simulink library "TOWER_MASTER"  (Simulink 8.8)
settings: Solver=ode45  StartTime=0.0  StopTime=10.0  RelTol=1e-3  EnableMultiTasking=on
undefined symbols (not defined in the file): AC, AC2THRESHOLD, BF_WD_MASTER, GAS_WD_MASTER, GASAC, SIXOSEM_F_WD_AC_MASTER
libraries: cdsEpicsOut x163, cdsFilt x111, cdsTP x68, cdsFiltCtrl x56, cdsEpicsIn x47, cdsMuxMatrix x14, cdsRms x14, TOWER_MASTER x11, STATE_BIO_MASTER x8, cdsEpicsBinIn x6, cdsFunctionCall x4, VIS_LIB x2
(part 18 of 19)

== system TOWER_MASTER/common_blocks/OKUTOMIGASMODAL/TEST ==
  Ground{1..5} (5 alike) : Ground
  M1 : cdsFilt/Subsystem  Tag=cdsFilt  Description=|
      | Purpose:                                                                                                                                                                                                                                  
      | Standard CDS IIR filter module.                                                                                                                                                                                                           
      |                                                                                                                                                                                                                                           
      | Operation:                                                                                                                                                                                                                                
      | Consists of 10 second order section IIR filters, plus a ramped gain stage. In FE code, also provides pre-defined test points and excitation channel inputs. The filter coefficients are defined in the LIGO system using the 'foton' tool.
      |                                                                                                                                                                                                                                           
      | Usage:                                                                                                                                                                                                                                    
      | Name the part with the desired filter module name.
      settings: AttributesFormatString=%<Tag>
  M2 : cdsFilt/Subsystem  Tag=cdsFilt  Description=|
      | Purpose:                                                                                                                                                                                                                                  
      | Standard CDS IIR filter module.                                                                                                                                                                                                           
      |                                                                                                                                                                                                                                           
      | Operation:                                                                                                                                                                                                                                
      | Consists of 10 second order section IIR filters, plus a ramped gain stage. In FE code, also provides pre-defined test points and excitation channel inputs. The filter coefficients are defined in the LIGO system using the 'foton' tool.
      |                                                                                                                                                                                                                                           
      | Usage:                                                                                                                                                                                                                                    
      | Name the part with the desired filter module name.
      settings: AttributesFormatString=%<Tag>
  M3 : cdsFilt/Subsystem  Tag=cdsFilt  Description=|
      | Purpose:                                                                                                                                                                                                                                  
      | Standard CDS IIR filter module.                                                                                                                                                                                                           
      |                                                                                                                                                                                                                                           
      | Operation:                                                                                                                                                                                                                                
      | Consists of 10 second order section IIR filters, plus a ramped gain stage. In FE code, also provides pre-defined test points and excitation channel inputs. The filter coefficients are defined in the LIGO system using the 'foton' tool.
      |                                                                                                                                                                                                                                           
      | Usage:                                                                                                                                                                                                                                    
      | Name the part with the desired filter module name.
      settings: AttributesFormatString=%<Tag>
  M4 : cdsFilt/Subsystem  Tag=cdsFilt  Description=|
      | Purpose:                                                                                                                                                                                                                                  
      | Standard CDS IIR filter module.                                                                                                                                                                                                           
      |                                                                                                                                                                                                                                           
      | Operation:                                                                                                                                                                                                                                
      | Consists of 10 second order section IIR filters, plus a ramped gain stage. In FE code, also provides pre-defined test points and excitation channel inputs. The filter coefficients are defined in the LIGO system using the 'foton' tool.
      |                                                                                                                                                                                                                                           
      | Usage:                                                                                                                                                                                                                                    
      | Name the part with the desired filter module name.
      settings: AttributesFormatString=%<Tag>
  M5 : cdsFilt/Subsystem  Tag=cdsFilt  Description=|
      | Purpose:                                                                                                                                                                                                                                  
      | Standard CDS IIR filter module.                                                                                                                                                                                                           
      |                                                                                                                                                                                                                                           
      | Operation:                                                                                                                                                                                                                                
      | Consists of 10 second order section IIR filters, plus a ramped gain stage. In FE code, also provides pre-defined test points and excitation channel inputs. The filter coefficients are defined in the LIGO system using the 'foton' tool.
      |                                                                                                                                                                                                                                           
      | Usage:                                                                                                                                                                                                                                    
      | Name the part with the desired filter module name.
      settings: AttributesFormatString=%<Tag>
  M1_Out : Outport
  M2_Out : Outport  Port=2
  M3_Out : Outport  Port=3
  M4_Out : Outport  Port=4
  M5_Out : Outport  Port=5
  wires:
  Ground5/1 -> M5/1
  Ground4/1 -> M4/1
  M4/1 -> M4_Out/1
  M5/1 -> M5_Out/1
  Ground3/1 -> M3/1
  Ground2/1 -> M2/1
  Ground1/1 -> M1/1
  M1/1 -> M1_Out/1
  M2/1 -> M2_Out/1
  M3/1 -> M3_Out/1

== system TOWER_MASTER/common_blocks/OKUTOMIKALMAN/ADD_OUTPUT ==
  D_In1 : Inport
  D_In2 : Inport  Port=2
  D_In3 : Inport  Port=3
  D_In4 : Inport  Port=4
  D_In5 : Inport  Port=5
  D_In6 : Inport  Port=6
  C_In1 : Inport  Port=7
  C_In2 : Inport  Port=8
  C_In3 : Inport  Port=9
  C_In4 : Inport  Port=10
  C_In5 : Inport  Port=11
  C_In6 : Inport  Port=12
  Sum{1..6} (6 alike) : Sum
  Xest_Out1 : Outport
  Xest_Out2 : Outport  Port=2
  Xest_Out3 : Outport  Port=3
  Xest_Out4 : Outport  Port=4
  Xest_Out5 : Outport  Port=5
  Xest_Out6 : Outport  Port=6
  wires:
  Sum1/1 -> Xest_Out1/1
  Sum2/1 -> Xest_Out2/1
  Sum3/1 -> Xest_Out3/1
  Sum4/1 -> Xest_Out4/1
  Sum5/1 -> Xest_Out5/1
  Sum6/1 -> Xest_Out6/1
  C_In1/1 -> Sum1/1
  C_In2/1 -> Sum2/1
  C_In3/1 -> Sum3/1
  C_In4/1 -> Sum4/1
  C_In6/1 -> Sum6/1
  C_In5/1 -> Sum5/1
  D_In1/1 -> Sum1/2
  D_In6/1 -> Sum6/2
  D_In5/1 -> Sum5/2
  D_In4/1 -> Sum4/2
  D_In3/1 -> Sum3/2
  D_In2/1 -> Sum2/2

== system TOWER_MASTER/common_blocks/OKUTOMIKALMAN/ADD_STATE ==
  B_In1 : Inport
  B_In2 : Inport  Port=2
  B_In3 : Inport  Port=3
  B_In4 : Inport  Port=4
  B_In5 : Inport  Port=5
  B_In6 : Inport  Port=6
  A_In1 : Inport  Port=7
  A_In2 : Inport  Port=8
  A_In3 : Inport  Port=9
  A_In4 : Inport  Port=10
  A_In5 : Inport  Port=11
  A_In6 : Inport  Port=12
  Sum{1..6} (6 alike) : Sum
  dX_Out1 : Outport
  dX_Out2 : Outport  Port=2
  dX_Out3 : Outport  Port=3
  dX_Out4 : Outport  Port=4
  dX_Out5 : Outport  Port=5
  dX_Out6 : Outport  Port=6
  wires:
  B_In2/1 -> Sum2/2
  B_In3/1 -> Sum3/2
  B_In4/1 -> Sum4/2
  B_In5/1 -> Sum5/2
  B_In6/1 -> Sum6/2
  B_In1/1 -> Sum1/2
  A_In5/1 -> Sum5/1
  A_In6/1 -> Sum6/1
  A_In4/1 -> Sum4/1
  A_In3/1 -> Sum3/1
  A_In2/1 -> Sum2/1
  A_In1/1 -> Sum1/1
  Sum6/1 -> dX_Out6/1
  Sum5/1 -> dX_Out5/1
  Sum4/1 -> dX_Out4/1
  Sum3/1 -> dX_Out3/1
  Sum2/1 -> dX_Out2/1
  Sum1/1 -> dX_Out1/1

== system TOWER_MASTER/common_blocks/OKUTOMIKALMAN/KEST ==
  X1_In : Inport
  X2_In : Inport  Port=2
  X3_In : Inport  Port=3
  X4_In : Inport  Port=4
  X5_In : Inport  Port=5
  X6_In : Inport  Port=6
  X1 : cdsFilt/Subsystem  Tag=cdsFilt  Description=|
      | Purpose:                                                                                                                                                                                                                                  
      | Standard CDS IIR filter module.                                                                                                                                                                                                           
      |                                                                                                                                                                                                                                           
      | Operation:                                                                                                                                                                                                                                
      | Consists of 10 second order section IIR filters, plus a ramped gain stage. In FE code, also provides pre-defined test points and excitation channel inputs. The filter coefficients are defined in the LIGO system using the 'foton' tool.
      |                                                                                                                                                                                                                                           
      | Usage:                                                                                                                                                                                                                                    
      | Name the part with the desired filter module name.
      settings: AttributesFormatString=%<Tag>
  X2 : cdsFilt/Subsystem  Tag=cdsFilt  Description=|
      | Purpose:                                                                                                                                                                                                                                  
      | Standard CDS IIR filter module.                                                                                                                                                                                                           
      |                                                                                                                                                                                                                                           
      | Operation:                                                                                                                                                                                                                                
      | Consists of 10 second order section IIR filters, plus a ramped gain stage. In FE code, also provides pre-defined test points and excitation channel inputs. The filter coefficients are defined in the LIGO system using the 'foton' tool.
      |                                                                                                                                                                                                                                           
      | Usage:                                                                                                                                                                                                                                    
      | Name the part with the desired filter module name.
      settings: AttributesFormatString=%<Tag>
  X3 : cdsFilt/Subsystem  Tag=cdsFilt  Description=|
      | Purpose:                                                                                                                                                                                                                                  
      | Standard CDS IIR filter module.                                                                                                                                                                                                           
      |                                                                                                                                                                                                                                           
      | Operation:                                                                                                                                                                                                                                
      | Consists of 10 second order section IIR filters, plus a ramped gain stage. In FE code, also provides pre-defined test points and excitation channel inputs. The filter coefficients are defined in the LIGO system using the 'foton' tool.
      |                                                                                                                                                                                                                                           
      | Usage:                                                                                                                                                                                                                                    
      | Name the part with the desired filter module name.
      settings: AttributesFormatString=%<Tag>
  X4 : cdsFilt/Subsystem  Tag=cdsFilt  Description=|
      | Purpose:                                                                                                                                                                                                                                  
      | Standard CDS IIR filter module.                                                                                                                                                                                                           
      |                                                                                                                                                                                                                                           
      | Operation:                                                                                                                                                                                                                                
      | Consists of 10 second order section IIR filters, plus a ramped gain stage. In FE code, also provides pre-defined test points and excitation channel inputs. The filter coefficients are defined in the LIGO system using the 'foton' tool.
      |                                                                                                                                                                                                                                           
      | Usage:                                                                                                                                                                                                                                    
      | Name the part with the desired filter module name.
      settings: AttributesFormatString=%<Tag>
  X5 : cdsFilt/Subsystem  Tag=cdsFilt  Description=|
      | Purpose:                                                                                                                                                                                                                                  
      | Standard CDS IIR filter module.                                                                                                                                                                                                           
      |                                                                                                                                                                                                                                           
      | Operation:                                                                                                                                                                                                                                
      | Consists of 10 second order section IIR filters, plus a ramped gain stage. In FE code, also provides pre-defined test points and excitation channel inputs. The filter coefficients are defined in the LIGO system using the 'foton' tool.
      |                                                                                                                                                                                                                                           
      | Usage:                                                                                                                                                                                                                                    
      | Name the part with the desired filter module name.
      settings: AttributesFormatString=%<Tag>
  X6 : cdsFilt/Subsystem  Tag=cdsFilt  Description=|
      | Purpose:                                                                                                                                                                                                                                  
      | Standard CDS IIR filter module.                                                                                                                                                                                                           
      |                                                                                                                                                                                                                                           
      | Operation:                                                                                                                                                                                                                                
      | Consists of 10 second order section IIR filters, plus a ramped gain stage. In FE code, also provides pre-defined test points and excitation channel inputs. The filter coefficients are defined in the LIGO system using the 'foton' tool.
      |                                                                                                                                                                                                                                           
      | Usage:                                                                                                                                                                                                                                    
      | Name the part with the desired filter module name.
      settings: AttributesFormatString=%<Tag>
  X1_Out : Outport
  X2_Out : Outport  Port=2
  X3_Out : Outport  Port=3
  X4_Out : Outport  Port=4
  X5_Out : Outport  Port=5
  X6_Out : Outport  Port=6
  wires:
  X2_In/1 -> X2/1
  X1_In/1 -> X1/1
  X6_In/1 -> X6/1
  X2/1 -> X2_Out/1
  X1/1 -> X1_Out/1
  X6/1 -> X6_Out/1
  X5_In/1 -> X5/1
  X4_In/1 -> X4/1
  X3_In/1 -> X3/1
  X5/1 -> X5_Out/1
  X4/1 -> X4_Out/1
  X3/1 -> X3_Out/1

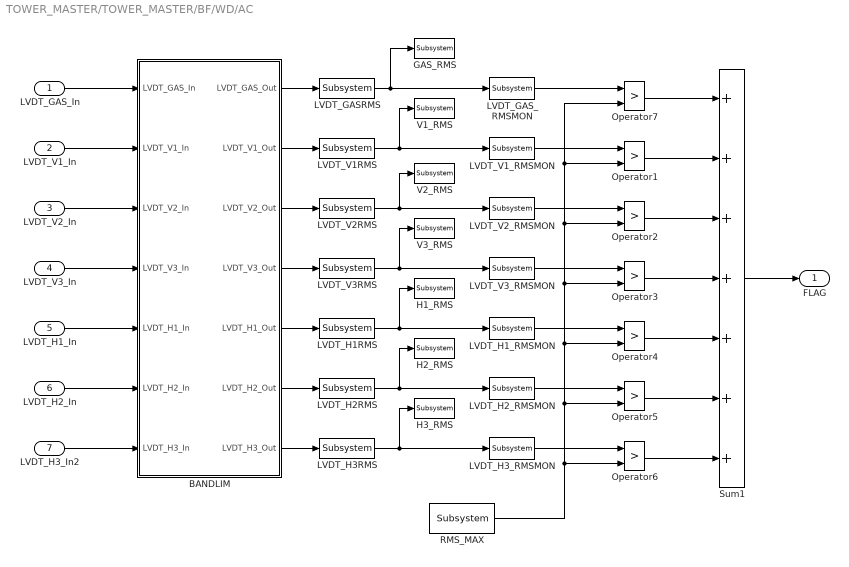
== system TOWER_MASTER/TOWER_MASTER/BF/WD/AC ==
  LVDT_GAS_In : Inport
  LVDT_V1_In : Inport  Port=2
  LVDT_V2_In : Inport  Port=3
  LVDT_V3_In : Inport  Port=4
  LVDT_H1_In : Inport  Port=5
  LVDT_H2_In : Inport  Port=6
  LVDT_H3_In2 : Inport  Port=7
  BANDLIM : Subsystem
  GAS_RMS : cdsTP/Subsystem  Tag=Test Point
      settings: AttributesFormatString=%<Tag>
  H1_RMS : cdsTP/Subsystem  Tag=Test Point
      settings: AttributesFormatString=%<Tag>
  H2_RMS : cdsTP/Subsystem  Tag=Test Point
      settings: AttributesFormatString=%<Tag>
  H3_RMS : cdsTP/Subsystem  Tag=Test Point
      settings: AttributesFormatString=%<Tag>
  LVDT_GASRMS : cdsRms/Subsystem  Tag=cdsRms  Description=|
      | Purpose:
      | Calculate an RMS based on the input signal.
      settings: AttributesFormatString=%<Tag>
  LVDT_GAS_RMSMON : cdsEpicsOut/Subsystem  Tag=cdsEpicsOutput  Description=|
      | Purpose:                                          
      | Output a FE signal to an EPICS channel.           
      |                                                   
      | Operation:                                        
      | Takes input value and passes it to EPICS record.  
      |                                                   
      | Usage:                                            
      | Name the part with the desired EPICS rrecord name.
      settings: AttributesFormatString=%<Tag>
  LVDT_H1RMS : cdsRms/Subsystem  Tag=cdsRms  Description=|
      | Purpose:
      | Calculate an RMS based on the input signal.
      settings: AttributesFormatString=%<Tag>
  LVDT_H1_RMSMON : cdsEpicsOut/Subsystem  Tag=cdsEpicsOutput  Description=|
      | Purpose:                                          
      | Output a FE signal to an EPICS channel.           
      |                                                   
      | Operation:                                        
      | Takes input value and passes it to EPICS record.  
      |                                                   
      | Usage:                                            
      | Name the part with the desired EPICS rrecord name.
      settings: AttributesFormatString=%<Tag>
  LVDT_H2RMS : cdsRms/Subsystem  Tag=cdsRms  Description=|
      | Purpose:
      | Calculate an RMS based on the input signal.
      settings: AttributesFormatString=%<Tag>
  LVDT_H2_RMSMON : cdsEpicsOut/Subsystem  Tag=cdsEpicsOutput  Description=|
      | Purpose:                                          
      | Output a FE signal to an EPICS channel.           
      |                                                   
      | Operation:                                        
      | Takes input value and passes it to EPICS record.  
      |                                                   
      | Usage:                                            
      | Name the part with the desired EPICS rrecord name.
      settings: AttributesFormatString=%<Tag>
  LVDT_H3RMS : cdsRms/Subsystem  Tag=cdsRms  Description=|
      | Purpose:
      | Calculate an RMS based on the input signal.
      settings: AttributesFormatString=%<Tag>
  LVDT_H3_RMSMON : cdsEpicsOut/Subsystem  Tag=cdsEpicsOutput  Description=|
      | Purpose:                                          
      | Output a FE signal to an EPICS channel.           
      |                                                   
      | Operation:                                        
      | Takes input value and passes it to EPICS record.  
      |                                                   
      | Usage:                                            
      | Name the part with the desired EPICS rrecord name.
      settings: AttributesFormatString=%<Tag>
  LVDT_V1RMS : cdsRms/Subsystem  Tag=cdsRms  Description=|
      | Purpose:
      | Calculate an RMS based on the input signal.
      settings: AttributesFormatString=%<Tag>
  LVDT_V1_RMSMON : cdsEpicsOut/Subsystem  Tag=cdsEpicsOutput  Description=|
      | Purpose:                                          
      | Output a FE signal to an EPICS channel.           
      |                                                   
      | Operation:                                        
      | Takes input value and passes it to EPICS record.  
      |                                                   
      | Usage:                                            
      | Name the part with the desired EPICS rrecord name.
      settings: AttributesFormatString=%<Tag>
  LVDT_V2RMS : cdsRms/Subsystem  Tag=cdsRms  Description=|
      | Purpose:
      | Calculate an RMS based on the input signal.
      settings: AttributesFormatString=%<Tag>
  LVDT_V2_RMSMON : cdsEpicsOut/Subsystem  Tag=cdsEpicsOutput  Description=|
      | Purpose:                                          
      | Output a FE signal to an EPICS channel.           
      |                                                   
      | Operation:                                        
      | Takes input value and passes it to EPICS record.  
      |                                                   
      | Usage:                                            
      | Name the part with the desired EPICS rrecord name.
      settings: AttributesFormatString=%<Tag>
  LVDT_V3RMS : cdsRms/Subsystem  Tag=cdsRms  Description=|
      | Purpose:
      | Calculate an RMS based on the input signal.
      settings: AttributesFormatString=%<Tag>
  LVDT_V3_RMSMON : cdsEpicsOut/Subsystem  Tag=cdsEpicsOutput  Description=|
      | Purpose:                                          
      | Output a FE signal to an EPICS channel.           
      |                                                   
      | Operation:                                        
      | Takes input value and passes it to EPICS record.  
      |                                                   
      | Usage:                                            
      | Name the part with the desired EPICS rrecord name.
      settings: AttributesFormatString=%<Tag>
  Operator{1,3..7} (6 alike) : RelationalOperator  Operator=>  OutDataTypeStr=boolean  RndMeth=Nearest
  Operator2 : RelationalOperator  Operator=>  OutDataTypeStr=boolean  ZeroCross=off  RndMeth=Nearest
  RMS_MAX : cdsEpicsIn/Subsystem  Tag=cdsEpicsIn  Description=|
      | Purpose:                                                                              
      | Create an EPICS input channel connection to the FE realtime controls.                 
      |                                                                                       
      | Operation:                                                                            
      | Outputs value from an EPICS ai record. Value is floating point with a precision of 3..
      |                                                                                       
      | Usage:                                                                                
      | Name the part with the desired EPICS channel name.
      settings: AttributesFormatString=%<Tag>
  Sum1 : Sum  Inputs=+++++++
  V1_RMS : cdsTP/Subsystem  Tag=Test Point
      settings: AttributesFormatString=%<Tag>
  V2_RMS : cdsTP/Subsystem  Tag=Test Point
      settings: AttributesFormatString=%<Tag>
  V3_RMS : cdsTP/Subsystem  Tag=Test Point
      settings: AttributesFormatString=%<Tag>
  FLAG : Outport
  wires:
  Operator7/1 -> Sum1/1
  Operator6/1 -> Sum1/7
  Operator5/1 -> Sum1/6
  Operator4/1 -> Sum1/5
  Operator3/1 -> Sum1/4
  Operator2/1 -> Sum1/3
  Operator1/1 -> Sum1/2
  LVDT_GAS_RMSMON/1 -> Operator7/1
  LVDT_GASRMS/1 -> LVDT_GAS_RMSMON/1, GAS_RMS/1
  BANDLIM/1(LVDT_GAS_Out) -> LVDT_GASRMS/1
  LVDT_H3_In2/1 -> BANDLIM/7(LVDT_H3_In)
  LVDT_H2_In/1 -> BANDLIM/6(LVDT_H2_In)
  LVDT_H1_In/1 -> BANDLIM/5(LVDT_H1_In)
  LVDT_V3_In/1 -> BANDLIM/4(LVDT_V3_In)
  LVDT_V2_In/1 -> BANDLIM/3(LVDT_V2_In)
  LVDT_V1_In/1 -> BANDLIM/2(LVDT_V1_In)
  LVDT_GAS_In/1 -> BANDLIM/1(LVDT_GAS_In)
  BANDLIM/7(LVDT_H3_Out) -> LVDT_H3RMS/1
  BANDLIM/6(LVDT_H2_Out) -> LVDT_H2RMS/1
  BANDLIM/5(LVDT_H1_Out) -> LVDT_H1RMS/1
  BANDLIM/4(LVDT_V3_Out) -> LVDT_V3RMS/1
  BANDLIM/3(LVDT_V2_Out) -> LVDT_V2RMS/1
  BANDLIM/2(LVDT_V1_Out) -> LVDT_V1RMS/1
  RMS_MAX/1 -> Operator1/2, Operator7/2, Operator2/2, Operator3/2, Operator4/2, Operator5/2, Operator6/2
  LVDT_V2RMS/1 -> V2_RMS/1, LVDT_V2_RMSMON/1
  LVDT_V1RMS/1 -> V1_RMS/1, LVDT_V1_RMSMON/1
  LVDT_V3RMS/1 -> V3_RMS/1, LVDT_V3_RMSMON/1
  LVDT_H1RMS/1 -> H1_RMS/1, LVDT_H1_RMSMON/1
  Sum1/1 -> FLAG/1
  LVDT_H2RMS/1 -> H2_RMS/1, LVDT_H2_RMSMON/1
  LVDT_H3RMS/1 -> H3_RMS/1, LVDT_H3_RMSMON/1
  LVDT_V1_RMSMON/1 -> Operator1/1
  LVDT_V2_RMSMON/1 -> Operator2/1
  LVDT_V3_RMSMON/1 -> Operator3/1
  LVDT_H1_RMSMON/1 -> Operator4/1
  LVDT_H2_RMSMON/1 -> Operator5/1
  LVDT_H3_RMSMON/1 -> Operator6/1

== system TOWER_MASTER/TOWER_MASTER/IP/WD/AC ==
  LVDT_H1_In : Inport
  LVDT_H2_In : Inport  Port=2
  LVDT_H3_In : Inport  Port=3
  ACC_H1_In : Inport  Port=4
  ACC_H2_In1 : Inport  Port=5
  ACC_H3_In1 : Inport  Port=6
  ACCH1RMS : cdsRms/Subsystem  Tag=cdsRms  Description=|
      | Purpose:
      | Calculate an RMS based on the input signal.
      settings: AttributesFormatString=%<Tag>
  ACCH1_RMS : cdsTP/Subsystem  Tag=Test Point
      settings: AttributesFormatString=%<Tag>
  ACCH2RMS : cdsRms/Subsystem  Tag=cdsRms  Description=|
      | Purpose:
      | Calculate an RMS based on the input signal.
      settings: AttributesFormatString=%<Tag>
  ACCH2_RMS : cdsTP/Subsystem  Tag=Test Point
      settings: AttributesFormatString=%<Tag>
  ACCH3RMS : cdsRms/Subsystem  Tag=cdsRms  Description=|
      | Purpose:
      | Calculate an RMS based on the input signal.
      settings: AttributesFormatString=%<Tag>
  ACCH3_RMS : cdsTP/Subsystem  Tag=Test Point
      settings: AttributesFormatString=%<Tag>
  ACC_H1_RMSMON : cdsEpicsOut/Subsystem  Tag=cdsEpicsOutput  Description=|
      | Purpose:                                          
      | Output a FE signal to an EPICS channel.           
      |                                                   
      | Operation:                                        
      | Takes input value and passes it to EPICS record.  
      |                                                   
      | Usage:                                            
      | Name the part with the desired EPICS rrecord name.
      settings: AttributesFormatString=%<Tag>
  ACC_H2_RMSMON : cdsEpicsOut/Subsystem  Tag=cdsEpicsOutput  Description=|
      | Purpose:                                          
      | Output a FE signal to an EPICS channel.           
      |                                                   
      | Operation:                                        
      | Takes input value and passes it to EPICS record.  
      |                                                   
      | Usage:                                            
      | Name the part with the desired EPICS rrecord name.
      settings: AttributesFormatString=%<Tag>
  ACC_H3_RMSMON : cdsEpicsOut/Subsystem  Tag=cdsEpicsOutput  Description=|
      | Purpose:                                          
      | Output a FE signal to an EPICS channel.           
      |                                                   
      | Operation:                                        
      | Takes input value and passes it to EPICS record.  
      |                                                   
      | Usage:                                            
      | Name the part with the desired EPICS rrecord name.
      settings: AttributesFormatString=%<Tag>
  BANDLIM : Subsystem
  LVDTH1RMS : cdsRms/Subsystem  Tag=cdsRms  Description=|
      | Purpose:
      | Calculate an RMS based on the input signal.
      settings: AttributesFormatString=%<Tag>
  LVDTH1_RMS : cdsTP/Subsystem  Tag=Test Point
      settings: AttributesFormatString=%<Tag>
  LVDTH2RMS : cdsRms/Subsystem  Tag=cdsRms  Description=|
      | Purpose:
      | Calculate an RMS based on the input signal.
      settings: AttributesFormatString=%<Tag>
  LVDTH2_RMS : cdsTP/Subsystem  Tag=Test Point
      settings: AttributesFormatString=%<Tag>
  LVDTH3RMS : cdsRms/Subsystem  Tag=cdsRms  Description=|
      | Purpose:
      | Calculate an RMS based on the input signal.
      settings: AttributesFormatString=%<Tag>
  LVDTH3_RMS : cdsTP/Subsystem  Tag=Test Point
      settings: AttributesFormatString=%<Tag>
  LVDT_H1_RMSMON : cdsEpicsOut/Subsystem  Tag=cdsEpicsOutput  Description=|
      | Purpose:                                          
      | Output a FE signal to an EPICS channel.           
      |                                                   
      | Operation:                                        
      | Takes input value and passes it to EPICS record.  
      |                                                   
      | Usage:                                            
      | Name the part with the desired EPICS rrecord name.
      settings: AttributesFormatString=%<Tag>
  LVDT_H2_RMSMON : cdsEpicsOut/Subsystem  Tag=cdsEpicsOutput  Description=|
      | Purpose:                                          
      | Output a FE signal to an EPICS channel.           
      |                                                   
      | Operation:                                        
      | Takes input value and passes it to EPICS record.  
      |                                                   
      | Usage:                                            
      | Name the part with the desired EPICS rrecord name.
      settings: AttributesFormatString=%<Tag>
  LVDT_H3_RMSMON : cdsEpicsOut/Subsystem  Tag=cdsEpicsOutput  Description=|
      | Purpose:                                          
      | Output a FE signal to an EPICS channel.           
      |                                                   
      | Operation:                                        
      | Takes input value and passes it to EPICS record.  
      |                                                   
      | Usage:                                            
      | Name the part with the desired EPICS rrecord name.
      settings: AttributesFormatString=%<Tag>
  Operator{1,3..6} (5 alike) : RelationalOperator  Operator=>  OutDataTypeStr=boolean  RndMeth=Nearest
  Operator2 : RelationalOperator  Operator=>  OutDataTypeStr=boolean  ZeroCross=off  RndMeth=Nearest
  RMS_MAX_ACC : cdsEpicsIn/Subsystem  Tag=cdsEpicsIn  Description=|
      | Purpose:                                                                              
      | Create an EPICS input channel connection to the FE realtime controls.                 
      |                                                                                       
      | Operation:                                                                            
      | Outputs value from an EPICS ai record. Value is floating point with a precision of 3..
      |                                                                                       
      | Usage:                                                                                
      | Name the part with the desired EPICS channel name.
      settings: AttributesFormatString=%<Tag>
  RMS_MAX_LVDT : cdsEpicsIn/Subsystem  Tag=cdsEpicsIn  Description=|
      | Purpose:                                                                              
      | Create an EPICS input channel connection to the FE realtime controls.                 
      |                                                                                       
      | Operation:                                                                            
      | Outputs value from an EPICS ai record. Value is floating point with a precision of 3..
      |                                                                                       
      | Usage:                                                                                
      | Name the part with the desired EPICS channel name.
      settings: AttributesFormatString=%<Tag>
  Sum1 : Sum  Inputs=++++++
  FLAG : Outport
  wires:
  RMS_MAX_LVDT/1 -> Operator1/2, Operator2/2, Operator3/2
  Operator6/1 -> Sum1/6
  Operator5/1 -> Sum1/5
  ACC_H3_RMSMON/1 -> Operator6/1
  ACC_H2_RMSMON/1 -> Operator5/1
  ACC_H1_RMSMON/1 -> Operator4/1
  LVDT_H3_RMSMON/1 -> Operator3/1
  LVDT_H2_RMSMON/1 -> Operator2/1
  LVDT_H1_RMSMON/1 -> Operator1/1
  ACCH3RMS/1 -> ACC_H3_RMSMON/1, ACCH3_RMS/1
  ACCH2RMS/1 -> ACC_H2_RMSMON/1, ACCH2_RMS/1
  Sum1/1 -> FLAG/1
  ACCH1RMS/1 -> ACC_H1_RMSMON/1, ACCH1_RMS/1
  LVDTH3RMS/1 -> LVDT_H3_RMSMON/1, LVDTH3_RMS/1
  LVDTH1RMS/1 -> LVDT_H1_RMSMON/1, LVDTH1_RMS/1
  LVDTH2RMS/1 -> LVDT_H2_RMSMON/1, LVDTH2_RMS/1
  RMS_MAX_ACC/1 -> Operator6/2, Operator5/2, Operator4/2
  Operator4/1 -> Sum1/4
  Operator3/1 -> Sum1/3
  Operator2/1 -> Sum1/2
  Operator1/1 -> Sum1/1
  LVDT_H1_In/1 -> BANDLIM/1(LVDT_H1_In)
  LVDT_H2_In/1 -> BANDLIM/2(LVDT_H2_In)
  LVDT_H3_In/1 -> BANDLIM/3(LVDT_H3_In)
  ACC_H1_In/1 -> BANDLIM/4(ACC_H1_In)
  ACC_H2_In1/1 -> BANDLIM/5(ACC_H2_In)
  ACC_H3_In1/1 -> BANDLIM/6(ACC_H3_In)
  BANDLIM/1(LVDT_H1_Out) -> LVDTH1RMS/1
  BANDLIM/2(LVDT_H2_Out) -> LVDTH2RMS/1
  BANDLIM/3(LVDT_H3_Out) -> LVDTH3RMS/1
  BANDLIM/4(ACC_H1_Out) -> ACCH1RMS/1
  BANDLIM/5(ACC_H2_Out) -> ACCH2RMS/1
  BANDLIM/6(ACC_H3_Out) -> ACCH3RMS/1

== system TOWER_MASTER/common_blocks/GASMASTER/WD/AC ==
  H1_In : Inport
  Abs1 : Abs
  BANDLIM : Subsystem
  GASRMS : cdsRms/Subsystem  Tag=cdsRms  Description=|
      | Purpose:
      | Calculate an RMS based on the input signal.
      settings: AttributesFormatString=%<Tag>
  GAS_RMS : cdsTP/Subsystem  Tag=Test Point
      settings: AttributesFormatString=%<Tag>
  GAS_RMSMON : cdsEpicsOut/Subsystem  Tag=cdsEpicsOutput  Description=|
      | Purpose:                                          
      | Output a FE signal to an EPICS channel.           
      |                                                   
      | Operation:                                        
      | Takes input value and passes it to EPICS record.  
      |                                                   
      | Usage:                                            
      | Name the part with the desired EPICS rrecord name.
      settings: AttributesFormatString=%<Tag>
  Operator1 : RelationalOperator  Operator=>  OutDataTypeStr=boolean  RndMeth=Nearest
  RMS_MAX : cdsEpicsIn/Subsystem  Tag=cdsEpicsIn  Description=|
      | Purpose:                                                                              
      | Create an EPICS input channel connection to the FE realtime controls.                 
      |                                                                                       
      | Operation:                                                                            
      | Outputs value from an EPICS ai record. Value is floating point with a precision of 3..
      |                                                                                       
      | Usage:                                                                                
      | Name the part with the desired EPICS channel name.
      settings: AttributesFormatString=%<Tag>
  FLAG : Outport
  wires:
  BANDLIM/1(H1_Out) -> GASRMS/1
  H1_In/1 -> BANDLIM/1(H1_In)
  GAS_RMSMON/1 -> Abs1/1
  Abs1/1 -> Operator1/1
  RMS_MAX/1 -> Operator1/2
  GASRMS/1 -> GAS_RMS/1, GAS_RMSMON/1
  Operator1/1 -> FLAG/1
